simulink model "INV_torque_command_limiter"  (R2025a)
settings: Solver=VariableStepAuto  StartTime=0.0  StopTime=10.0  RelTol=1e-3
settings Model: Creator=taiji  LastModifiedBy=taiji

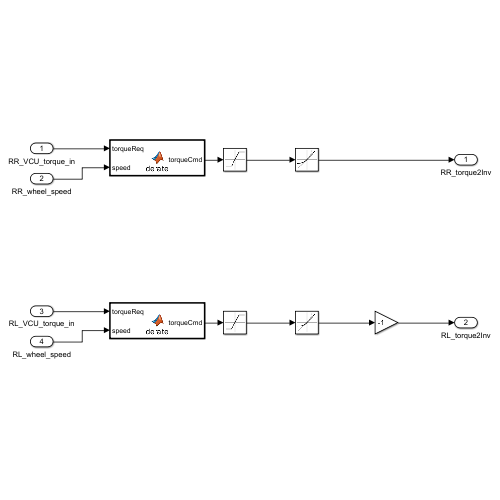
[thumbnail: Simulink's stored preview of the top-level diagram]
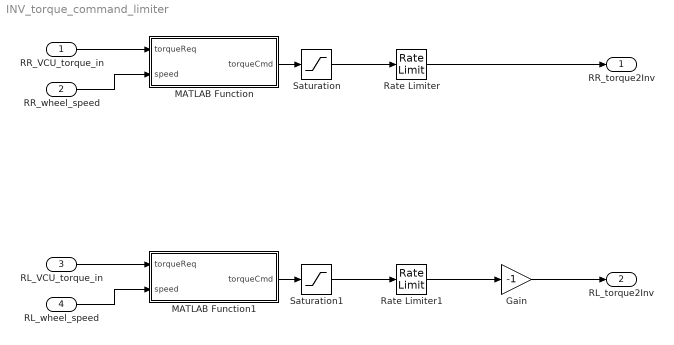
== system INV_torque_command_limiter ==
  RR_VCU_torque_in : Inport
  RR_wheel_speed : Inport  Port=2
  RL_VCU_torque_in : Inport  Port=3
  RL_wheel_speed : Inport  Port=4
  Gain : Gain  Gain=-1
  MATLAB Function : MATLAB Function  TreatAsAtomicUnit=on
  MATLAB Function1 : MATLAB Function  TreatAsAtomicUnit=on
  Rate Limiter : RateLimiter  RisingSlewLimit=4  FallingSlewLimit=-4
  Rate Limiter1 : RateLimiter  RisingSlewLimit=4  FallingSlewLimit=-4
  Saturation : Saturate  UpperLimit=10  LowerLimit=0
  Saturation1 : Saturate  UpperLimit=10  LowerLimit=0
  RR_torque2Inv : Outport
  RL_torque2Inv : Outport  Port=2
  wires:
  Saturation/1 -> Rate Limiter/1
  Saturation1/1 -> Rate Limiter1/1
  Rate Limiter1/1 -> Gain/1
  MATLAB Function/1(torqueCmd) -> Saturation/1
  MATLAB Function1/1(torqueCmd) -> Saturation1/1
  Gain/1 -> RL_torque2Inv/1
  Rate Limiter/1 -> RR_torque2Inv/1
  RR_VCU_torque_in/1 -> MATLAB Function/1(torqueReq)
  RR_wheel_speed/1 -> MATLAB Function/2(speed)
  RL_VCU_torque_in/1 -> MATLAB Function1/1(torqueReq)
  RL_wheel_speed/1 -> MATLAB Function1/2(speed)

== matlab function INV_torque_command_limiter/MATLAB Function ==
  data: torqueReq input; torqueCmd output; speed input
function torqueCmd  = derate(torqueReq, speed)

if speed < 230
    torqueCmd = torqueReq;
else
    torqueCmd = torqueReq*(1-(speed-230)/370);
end

== matlab function INV_torque_command_limiter/MATLAB Function1 ==
  data: torqueReq input; torqueCmd output; speed input
function torqueCmd  = derate(torqueReq, speed)

if speed < 230
    torqueCmd = torqueReq;
else
    torqueCmd = torqueReq*(1-(speed-230)/370);
end
